simulink model "intel_motor_control_rl2freddie"  (Simulink 10.3)
settings: Solver=FixedStepDiscrete  StartTime=0.0  StopTime=0.7  FixedStep=62.5e-6 % 16 kHz  RelTol=1e-3  EnableMultiTasking=on
undefined symbols (not defined in the file or in its folder): DiscIntNeverNeededParam, I_max, Position_PI_Limit
libraries: simulink x9, dspsrcs4 x2, rllib x1
(part 1 of 2)
settings Model: Creator=tchau  LastModifiedBy=ludwigjonsson  MultithreadedSim=on
settings Model: SuppressorTable=|
  | <?xml version="1.0" encoding="UTF-8" standalone="yes" ?>
  | <!DOCTYPE boost_serialization>
  | <boost_serialization signature="serialization::archive" version="17">
  | <DiagnosticSuppressor class_id="0" tracking_level="0" version="7">
  | 	<Table class_id="1" tracking_level="0" version="0">
  | 		<count>1</count>
  | 		<bucket_count>2</bucket_count>
  | 		<item_version>0</item_version>
  | 		<item class_id="2" tracking_level="0" version="0">
  | 			<first class_id="3" tracking_level="0" version="7">
  | 				<Source class_id="4" tracking_level="0" version="0">
  | 					<count>1</count>
  | 					<item_version>0</item_version>
  | 					<item>7415:2</item>
  | 				</Source>
  | 			</first>
  | 			<second class_id="5" tracking_level="0" version="7">
  | 				<SuppressedData class_id="6" tracking_level="0" version="0">
  | 					<count>2</count>
  | 					<bucket_count>2</bucket_count>
  | 					<item_version>0</item_version>
  | 					<item class_id="7" tracking_level="0" version="0">
  | 						<first class_id="8" tracking_level="0" version="7">
  | 							<ID>Simulink:DataType:WarningOverFlowDetected</ID>
  | 							<Cause>
  | 								<Source>
  | 									<count>0</count>
  | 									<item_version>0</item_version>
  | 								</Source>
  | 							</Cause>
  | 						</first>
  | 						<second class_id="9" tracking_level="0" version="7">
  | 							<Comment></Comment>
  | 							<User></User>
  | 							<LastModified class_id="10" tracking_level="0" version="0">
  | 								<ptime_date class_id="11" tracking_level="0" version="0">
  | 									<date>20160608</date>
  | 								</ptime_date>
  | 								<ptime_time_duration class_id="12" tracking_level="0" version="1">
  | 									<is_special>0</is_special>
  | 									<time_duration_hours>15</time_duration_hours>
  | 									<time_duration_minutes>23</time_duration_minutes>
  | 									<time_duration_seconds>17</time_duration_seconds>
  | 									<time_duration_fractional_seconds>0</time_duration_fractional_seconds>
  | 								</ptime_time_duration>
  | 							</LastModified>
  | 							<SuppressionType>1</SuppressionType>
  | 						</second>
  | 					</item>
  | 					<item>
  | 						<first>
  | 							<ID>SimulinkFixedPoint:util:Overflowoccurred</ID>
  | 							<Cause>
  | 								<Source>
  | 									<count>0</count>
  | 									<item_version>0</item_version>
  | 								</Source>
  | 							</Cause>
  | 						</first>
  | 						<second>
  | 							<Comment></Comment>
  | 							<User></User>
  | 							<LastModified>
  | 								<ptime_date>
  | 									<date>20160608</date>
  | 								</ptime_date>
  | 								<ptime_time_duration>
  | 									<is_special>0</is_special>
  | 									<time_duration_hours>15</time_duration_hours>
  | 									<time_duration_minutes>23</time_duration_minutes>
  | 									<time_duration_seconds>17</time_duration_seconds>
  | 									<time_duration_fractional_seconds>0</time_duration_fractional_seconds>
  | 								</ptime_time_duration>
  | 							</LastModified>
  | 							<SuppressionType>1</SuppressionType>
  | 						</second>
  | 					</item>
  | 				</SuppressedData>
  | 			</second>
  | 		</item>
  | 	</Table>
  | </DiagnosticSuppressor>
  | 
  | </boost_serialization>
  | 
  | </boost_serialization>
settings DataIOCC: SignalLoggingSaveFormat=Dataset  SaveOutput=off  SignalLogging=off  DSMLogging=off  SaveTime=off  ReturnWorkspaceOutputs=on
settings OptimizationCC: BlockReduction=off  ConditionallyExecuteInputs=off  DefaultParameterBehavior=Inlined  InlineInvariantSignals=on  ExpressionDepthLimit=128  EfficientFloat2IntCast=on  SimCompilerOptimization=on
settings DebuggingCC: AlgebraicLoopMsg=error  UnderspecifiedInitializationDetection=Simplified  MergeDetectMultiDrivingBlocksExec=error  SolverPrmCheckMsg=warning  SingleTaskRateTransMsg=error  FcnCallInpInsideContextMsg=error  StateNameClashWarn=none
settings HardwareCC: ProdHWDeviceType=ASIC/FPGA->ASIC/FPGA  TargetBitPerLong=64  TargetBitPerPointer=64  TargetBitPerSizeT=64  TargetBitPerPtrDiffT=64  TargetLongLongMode=on  TargetIntDivRoundTo=Zero  TargetEndianess=LittleEndian  TargetWordSize=64  TargetHWDeviceType=MATLAB Host  ProdEqTarget=off
settings GRTTargetCC: CombineOutputUpdateFcns=on  MatFileLogging=off  SupportNonFinite=off  GRTInterface=off

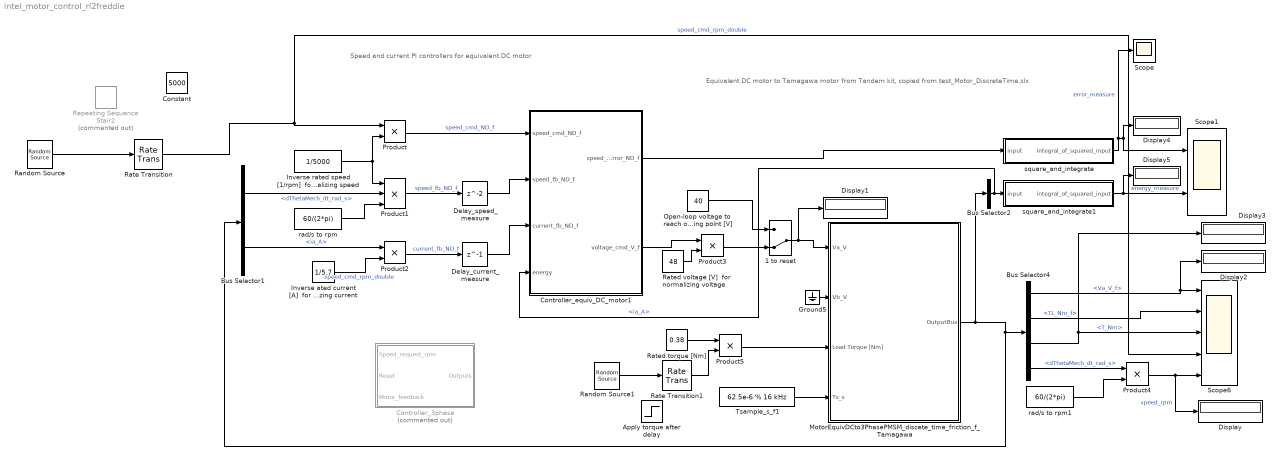
== system intel_motor_control_rl2freddie ==
  note: Equivalent DC motor to Tamagawa motor from Tandem kit,
      | copied from test_Motor_DiscreteTime.slx
  note: Speed and current PI controllers
      | for equivalent DC motor
  1 to reset : ManualSwitch  CurrentSetting=0
  "Apply torque after delay " : Step  Time=0.05  SampleTime=0
  Bus Selector1 : BusSelector  OutputSignals=dThetaMech_dt_rad_s,ia_A
  Bus Selector2 : BusSelector  OutputSignals=ia_A
  Bus Selector4 : BusSelector  OutputSignals=Va_V_f,TL_Nm_f,T_Nm,dThetaMech_dt_rad_s
  Constant : Constant  Value=5000
  Controller_3phase : Subsystem  Commented=on
  Controller_equiv_DC_motor1 : Subsystem
  Delay_current_measure : Delay  DelayLength=1  InitialCondition=0
  Delay_speed_measure : Delay  InitialCondition=0
  Display{,1..5} (6 alike) : Display
  Ground5 : Ground
  Inverse ated current [A]  for normalizing current : Constant  Value=1/5.7  OutDataTypeStr=double
  Inverse rated speed [1/rpm]  for normalizing speed : Constant  Value=1/5000  OutDataTypeStr=double
  MotorEquivDCto3PhasePMSM_discete_time_friction_f_Tamagawa : Subsystem  mask(Intel PMSM equiv DC){R_ohm=0.68/3, L_H=3e-3/3, Ke_Vs_rad=0.07, Kt_Nm_A=0.07, PolePairs_int=2, J_kgm2=0.165e-4, Tf_Nm=0.02}
      mask prompts: R_ohm "Phase resistance [Ohm]"; L_H "Phase inductance [H]"; Ke_Vs_rad "Back-emf constant kE, based on peak phase values [Vs/rad]"; Kt_Nm_A "Motor torque constant kT, based on peak phase values [Nm/A]"; PolePairs_int "Number of pole pairs (0.5*n poles)  [integer]"; J_kgm2 "Mechanical inertia [kgm^2]"; Tf_Nm "Static friction Tf [Nm]"
      mask help: Intel motor model, equiv DC to PMSM
  Open-loop voltage to  reach operating point [V] : Constant  Value=40  OutDataTypeStr=double
  Product{,2..5} (5 alike) : Product
  Product1 : Product  Inputs=***
  Random Source : dspsrcs4/Random Source  SrcType=Uniform  NormMethod=Ziggurat  CltLength=12  MinVal=-5000  MaxVal=5000  MeanVal=0  VarVal=1  RepMode=Specify seed  rawSeed=randSeed  IsInherit=off  SampMode=Discrete  SampTime=650*62.5e-6  SampFrame=1  DataType=Double  OutComplex=Real  OutputFrames=off
  Random Source1 : dspsrcs4/Random Source  SrcType=Uniform  NormMethod=Ziggurat  CltLength=12  MinVal=-1  MaxVal=1  MeanVal=0  VarVal=1  RepMode=Specify seed  rawSeed=randSeed  IsInherit=off  SampMode=Discrete  SampTime=450*62.5e-6  SampFrame=1  DataType=Double  OutComplex=Real  OutputFrames=off
  Rate Transition : RateTransition  OutPortSampleTime=62.5e-6
  Rate Transition1 : RateTransition  OutPortSampleTime=62.5e-6
  Rated torque [Nm] : Constant  Value=0.38  OutDataTypeStr=double
  Rated voltage [V]  for normalizing voltage : Constant  Value=48  OutDataTypeStr=double
  Repeating Sequence Stair2 : simulink/Sources/Repeating Sequence Stair  Commented=on  OutValues=(rand(200,1)-0.5)*10000  tsamp=500*62.5e-6  OutMin=[]  OutMax=[]  OutDataTypeStr=double  OutputDataTypeScalingMode=double  OutDataType=fixdt(0,8)  ConRadixGroup=Best Precision: Vector-wise  OutScaling=2^-12
  Scope : Scope
  Scope1 : Scope  NumInputPorts=2
  Scope6 : Scope  NumInputPorts=5
  Tsample_s_f1 : Constant  Value=62.5e-6 % 16 kHz  OutDataTypeStr=double
  rad/s to rpm : Constant  Value=60/(2*pi)  OutDataTypeStr=double
  rad/s to rpm1 : Constant  Value=60/(2*pi)  OutDataTypeStr=double
  square_and_integrate : Subsystem
  square_and_integrate1 : Subsystem
  wires:
  Rate Transition/1 -> Scope6/4, Product/1  "speed_cmd_rpm_double"
  MotorEquivDCto3PhasePMSM_discete_time_friction_f_Tamagawa/1(OutputBus) -> Bus Selector2/1, Bus Selector1/1, Bus Selector4/1
  Bus Selector4/3 -> Scope6/3, Display3/1  "<T_Nm>"
  Ground5/1 -> MotorEquivDCto3PhasePMSM_discete_time_friction_f_Tamagawa/2(Vb_V)
  Bus Selector4/1 -> Display2/1, Scope6/1  "<Va_V_f>"
  Product5/1 -> MotorEquivDCto3PhasePMSM_discete_time_friction_f_Tamagawa/3(Load Torque [Nm])
  Bus Selector4/4 -> Product4/1  "<dThetaMech_dt_rad_s>"
  Product/1 -> Controller_equiv_DC_motor1/1(speed_cmd_ND_f)  "speed_cmd_ND_f"
  Tsample_s_f1/1 -> MotorEquivDCto3PhasePMSM_discete_time_friction_f_Tamagawa/4(Ts_s)
  Inverse rated speed [1/rpm]  for normalizing speed/1 -> Product1/1, Product/2
  Product1/1 -> Delay_speed_measure/1  "speed_fb_ND_f"
  Bus Selector1/1 -> Product1/2  "<dThetaMech_dt_rad_s>"
  Bus Selector1/2 -> Product2/1  "<ia_A>"
  Inverse ated current [A]  for normalizing current/1 -> Product2/2  "speed_cmd_rpm_double"
  Controller_equiv_DC_motor1/2(voltage_cmd_V_f) -> Product3/1
  Rated voltage [V]  for normalizing voltage/1 -> Product3/2
  rad/s to rpm/1 -> Product1/3
  Product2/1 -> Delay_current_measure/1  "current_fb_ND_f"
  Product4/1 -> Scope6/5, Display/1  "speed_rpm"
  rad/s to rpm1/1 -> Product4/2
  Open-loop voltage to  reach operating point [V]/1 -> 1 to reset/1
  Product3/1 -> 1 to reset/2
  1 to reset/1 -> Display1/1, MotorEquivDCto3PhasePMSM_discete_time_friction_f_Tamagawa/1(Va_V)
  Rated torque [Nm]/1 -> Product5/1
  Bus Selector4/2 -> Scope6/2  "<TL_Nm_f>"
  Controller_equiv_DC_motor1/1(speed_error_ND_f) -> square_and_integrate/1(input)
  square_and_integrate/1(integral_of_squared_input) -> Scope/1, Scope1/1, Display4/1  "error_measure"
  Bus Selector2/1 -> Controller_equiv_DC_motor1/4(energy), square_and_integrate1/1(input)  "<ia_A>"
  square_and_integrate1/1(integral_of_squared_input) -> Display5/1, Scope1/2  "energy_measure"
  Delay_speed_measure/1 -> Controller_equiv_DC_motor1/2(speed_fb_ND_f)
  Delay_current_measure/1 -> Controller_equiv_DC_motor1/3(current_fb_ND_f)
  Random Source1/1 -> Rate Transition1/1
  Random Source/1 -> Rate Transition/1
  Rate Transition1/1 -> Product5/2

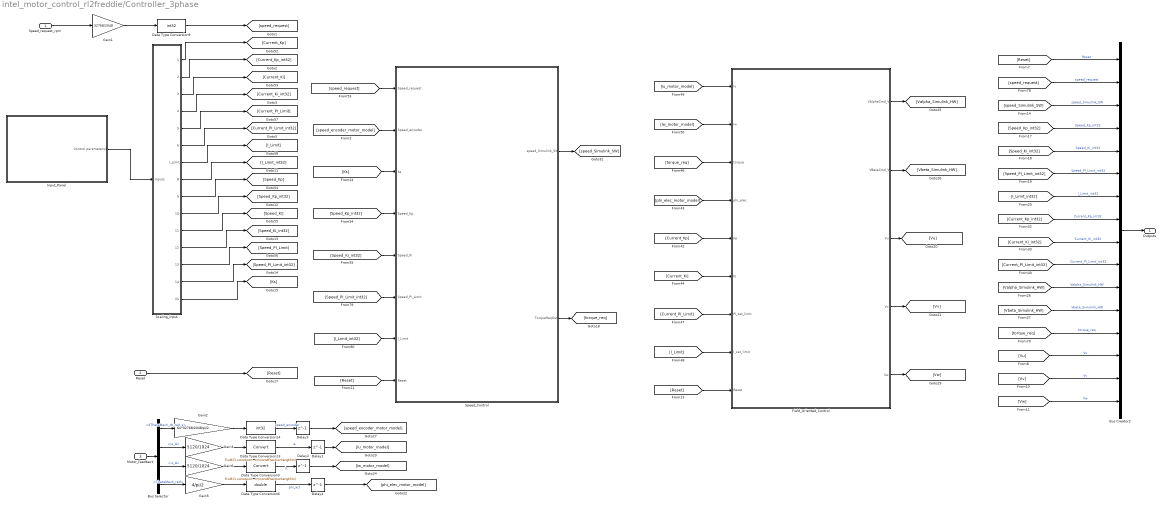
== system intel_motor_control_rl2freddie/Controller_3phase ==
  Speed_request_rpm : Inport
  Reset : Inport  Port=2  PortDimensions=1
  Motor_feedback : Inport  Port=3
  Bus Creator2 : BusCreator  Inputs=16
  Bus Selector : BusSelector  OutputSignals=dThetaMech_dt_rad_s,ia_A,ic_A,ThetaMech_rad
  Data Type Conversion13 : DataTypeConversion  OutDataTypeStr=fixdt(1,constwordlengthIn,constfractionlengthIn)
  Data Type Conversion14 : DataTypeConversion  OutDataTypeStr=int32
  Data Type Conversion3 : DataTypeConversion  OutDataTypeStr=fixdt(1,constwordlengthIn,constfractionlengthIn)
  Data Type Conversion6 : DataTypeConversion  OutDataTypeStr=double
  Data Type Conversion9 : DataTypeConversion  OutDataTypeStr=int32
  Delay{1..4} (4 alike) : Delay  DelayLength=1  InitialCondition=0
  Field_Oriented_Control : Subsystem
  Gain1 : Gain  Gain=32768/2048
  Gain2 : Gain  Gain=60*32768/2048/pi/2  OutDataTypeStr=single
  Gain3 : Gain  Gain=5120/1024  OutDataTypeStr=single
  Gain5 : Gain  Gain=4/pi/2  OutDataTypeStr=single
  Gain6 : Gain  Gain=5120/1024  OutDataTypeStr=single
  Input_Panel : Subsystem
      mask Display: fprintf('Setup\nParameters')
  Scaling_input : Subsystem
  Speed_Control : Subsystem
  Outputs : Outport
  wires:
  Data Type Conversion9/1 -> [speed_request]
  Speed_request_rpm/1 -> Gain1/1
  Gain1/1 -> Data Type Conversion9/1
  Input_Panel/1(Control parameters1) -> Scaling_input/1(Inputs)
  Field_Oriented_Control/2(VBetaCmd_V) -> [Vbeta_Simulink_HW]
  Field_Oriented_Control/1(VAlphaCmd_V) -> [Valpha_Simulink_HW]
  Data Type Conversion3/1 -> Delay2/1  "ic"
  Gain6/1 -> Data Type Conversion3/1
  Data Type Conversion13/1 -> Delay1/1  "ia"
  Gain3/1 -> Data Type Conversion13/1
  Data Type Conversion6/1 -> Delay4/1  "phi_act"
  Gain5/1 -> Data Type Conversion6/1
  Data Type Conversion14/1 -> Delay3/1  "speed_encoder"
  Gain2/1 -> Data Type Conversion14/1
  [Vw] -> Bus Creator2/16  "Vw"
  [Vv] -> Bus Creator2/15  "Vv"
  [Vu] -> Bus Creator2/14  "Vu"
  Field_Oriented_Control/5(Vw) -> [Vw]
  Bus Selector/2 -> Gain3/1  "<ia_A>"
  Bus Selector/4 -> Gain5/1  "<ThetaMech_rad>"
  Bus Selector/1 -> Gain2/1  "<dThetaMech_dt_rad_s>"
  Delay3/1 -> [speed_encoder_motor_model]
  Bus Selector/3 -> Gain6/1  "<ic_A>"
  Delay4/1 -> [phi_elec_motor_model]
  Delay2/1 -> [Iw_motor_model]
  Delay1/1 -> [Iu_motor_model]
  [speed_encoder_motor_model] -> Speed_Control/2(Speed_encoder)
  Motor_feedback/1 -> Bus Selector/1
  Field_Oriented_Control/4(Vv) -> [Vv]
  Field_Oriented_Control/3(Vu) -> [Vu]
  [Reset] -> Field_Oriented_Control/9(Reset)
  [I_Limit] -> Field_Oriented_Control/8(I_sat_limit)
  [Current_PI_Limit] -> Field_Oriented_Control/7(PI_sat_limit)
  [Current_Ki] -> Field_Oriented_Control/6(Ki)
  [Current_Kp] -> Field_Oriented_Control/5(Kp)
  [phi_elec_motor_model] -> Field_Oriented_Control/4(phi_elec)
  [torque_req] -> Field_Oriented_Control/3(torque)
  [Iw_motor_model] -> Field_Oriented_Control/2(Iw)
  [Iu_motor_model] -> Field_Oriented_Control/1(Iu)
  [torque_req] -> Bus Creator2/13  "torque_req"
  [Vbeta_Simulink_HW] -> Bus Creator2/12  "Vbeta_Simulink_HW"
  [Valpha_Simulink_HW] -> Bus Creator2/11  "Valpha_Simulink_HW"
  Bus Creator2/1 -> Outputs/1
  [Reset] -> Bus Creator2/1  "Reset"
  [Current_PI_Limit_int32] -> Bus Creator2/10  "Current_PI_Limit_int32"
  [Current_Ki_int32] -> Bus Creator2/9  "Current_Ki_int32"
  [Current_Kp_int32] -> Bus Creator2/8  "Current_Kp_int32"
  [I_Limit_int32] -> Bus Creator2/7  "I_Limit_int32"
  [Speed_PI_Limit_int32] -> Bus Creator2/6  "Speed_PI_Limit_int32"
  [Speed_Ki_int32] -> Bus Creator2/5  "Speed_Ki_int32"
  [Speed_Kp_int32] -> Bus Creator2/4  "Speed_Kp_int32"
  [I_Limit_int32] -> Speed_Control/7(I_Limit)
  [Speed_PI_Limit_int32] -> Speed_Control/6(Speed_PI_Limit)
  [Speed_Ki_int32] -> Speed_Control/5(Speed_Ki)
  [Speed_Kp_int32] -> Speed_Control/4(Speed_Kp)
  [speed_request] -> Speed_Control/1(Speed_request)
  Scaling_input/15(Ks) -> [Ks]
  Scaling_input/14(Speed_PI_Limit_int32) -> [Speed_PI_Limit_int32]
  Scaling_input/13(Speed_PI_Limit) -> [Speed_PI_Limit]
  Scaling_input/12(Speed_Ki_int32) -> [Speed_Ki_int32]
  Scaling_input/11(Speed_Ki) -> [Speed_Ki]
  Scaling_input/10(Speed_Kp_int32) -> [Speed_Kp_int32]
  Scaling_input/9(Speed_Kp) -> [Speed_Kp]
  Scaling_input/8(I_Limit_int32) -> [I_Limit_int32]
  Scaling_input/7(I_Limit) -> [I_Limit]
  Scaling_input/6(Current_PI_Limit_int32) -> [Current_PI_Limit_int32]
  Scaling_input/5(Current_PI_Limit) -> [Current_PI_Limit]
  Scaling_input/4(Current_Ki_int32) -> [Current_Ki_int32]
  Scaling_input/3(Current_Ki) -> [Current_Ki]
  Scaling_input/2(Current_Kp_int32) -> [Current_Kp_int32]
  Scaling_input/1(Current_Kp) -> [Current_Kp]
  [speed_request] -> Bus Creator2/2  "speed_request"
  Reset/1 -> [Reset]
  [speed_Simulink_SW] -> Bus Creator2/3  "speed_Simulink_SW"
  [Ks] -> Speed_Control/3(Ks)
  [Reset] -> Speed_Control/8(Reset)
  Speed_Control/1(speed_Simulink_SW) -> [speed_Simulink_SW]
  Speed_Control/2(TorqueReqOut) -> [torque_req]

== system intel_motor_control_rl2freddie/Controller_equiv_DC_motor1 ==
  note: RL Controller
  speed_cmd_ND_f : Inport
  speed_fb_ND_f : Inport  Port=2  PortDimensions=1
  current_fb_ND_f : Inport  Port=3  PortDimensions=1
  energy : Inport  Port=4
  1 to reset : ManualSwitch
  FALSE_bool : Constant  Value=0  OutDataTypeStr=boolean
  PI_Ctrl_float_speed : Subsystem
  TRUE_bool : Constant  OutDataTypeStr=boolean
  abs_limit_output_ND_f : Constant  OutDataTypeStr=double
  speed_error_ND_f : Outport
  voltage_cmd_V_f : Outport  Port=2
  wires:
  speed_cmd_ND_f/1 -> PI_Ctrl_float_speed/1(cmd_f)
  speed_fb_ND_f/1 -> PI_Ctrl_float_speed/2(fb_f)
  abs_limit_output_ND_f/1 -> PI_Ctrl_float_speed/3(output_abs_limit_f)
  current_fb_ND_f/1 -> PI_Ctrl_float_speed/6(Icurrent_fb)
  1 to reset/1 -> PI_Ctrl_float_speed/4(Reset_bool)
  FALSE_bool/1 -> 1 to reset/1
  TRUE_bool/1 -> 1 to reset/2
  PI_Ctrl_float_speed/1(error_f) -> speed_error_ND_f/1  "speed_error_ND_f"
  energy/1 -> PI_Ctrl_float_speed/5(energy)
  PI_Ctrl_float_speed/2(output_f) -> voltage_cmd_V_f/1

== system intel_motor_control_rl2freddie/MotorEquivDCto3PhasePMSM_discete_time_friction_f_Tamagawa ==
  Va_V : Inport
  Vb_V : Inport  Port=2
  Load Torque [Nm] : Inport  Port=3
  Ts_s : Inport  Port=4
  Bus Creator1 : BusCreator  Inputs=7
  Load Torque [Nm]1 : InportShadow  Port=3
  Motor electromagnetic : Subsystem
  Motor mechanical : Subsystem  mask(Inertia){J_kgm2=J_kgm2}
      mask prompts: J_kgm2 "Inertia [kgm^2]"
      mask help:
      | Mechanical inertia with two attachment points A and B.
      | Torque is applied to the inertia from side A and side B.
      | The combined torque acting on the inertia produces acceleration,
      | velocity and displacement. Velocity and displacement are output as these
      | are the states of the system.
  Ts_s1 : InportShadow  Port=4
  Va_V1 : InportShadow
  Vb_V1 : InportShadow  Port=2
  OutputBus : Outport
  wires:
  Ts_s1/1 -> Motor electromagnetic/4(Ts_s)
  Motor mechanical/1(dTheta_dt_rad_s) -> Motor electromagnetic/3(dThetaMech_dt_rad_s), Bus Creator1/6  "dThetaMech_dt_rad_s"
  Ts_s/1 -> Motor mechanical/3(Ts_s)
  Load Torque [Nm]/1 -> Motor mechanical/2(TB_Nm)  "TL_Nm_f"
  Va_V/1 -> Motor electromagnetic/1(Va_V)  "Va_V_f"
  Bus Creator1/1 -> OutputBus/1
  Vb_V/1 -> Motor electromagnetic/2(Vb_V)  "Vb_V_f"
  Va_V1/1 -> Bus Creator1/1  "Va_V_f"
  Vb_V1/1 -> Bus Creator1/2  "Vb_V_f"
  Motor electromagnetic/1(ia_A) -> Bus Creator1/4  "ia_A"
  Motor electromagnetic/2(T_Nm) -> Motor mechanical/1(TA_Nm), Bus Creator1/5  "T_Nm"
  Motor mechanical/2(Theta_rad) -> Bus Creator1/7  "ThetaMech_rad"
  Load Torque [Nm]1/1 -> Bus Creator1/3  "TL_Nm_f"

== system intel_motor_control_rl2freddie/square_and_integrate ==
  input : Inport
  Add : Sum
  Product6 : Product  Inputs=***
  Tsample_s_f2 : Constant  Value=62.5e-6 % 16 kHz  OutDataTypeStr=double
  delay_to_integrate : Delay  DelayLength=1  InitialCondition=0
  integral_of_squared_input : Outport
  wires:
  delay_to_integrate/1 -> integral_of_squared_input/1, Add/2
  Product6/1 -> Add/1
  Tsample_s_f2/1 -> Product6/3
  Add/1 -> delay_to_integrate/1
  input/1 -> Product6/1, Product6/2

== system intel_motor_control_rl2freddie/square_and_integrate1 ==
  input : Inport
  Add : Sum
  Product6 : Product  Inputs=***
  Tsample_s_f2 : Constant  Value=62.5e-6 % 16 kHz  OutDataTypeStr=double
  delay_to_integrate : Delay  DelayLength=1  InitialCondition=0
  integral_of_squared_input : Outport
  wires:
  input/1 -> Product6/2, Product6/1
  Add/1 -> delay_to_integrate/1
  Tsample_s_f2/1 -> Product6/3
  Product6/1 -> Add/1
  delay_to_integrate/1 -> Add/2, integral_of_squared_input/1

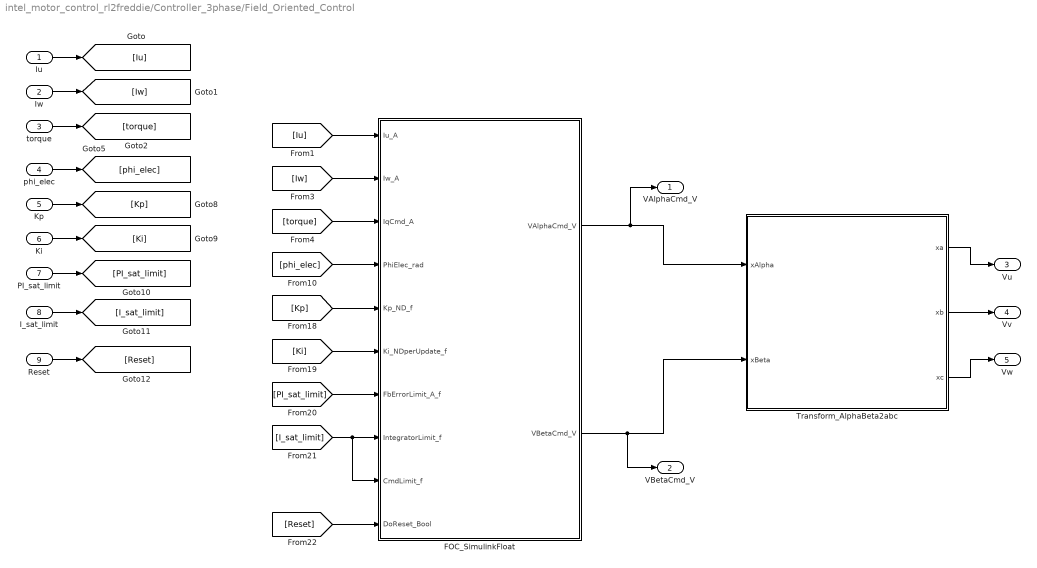
== system intel_motor_control_rl2freddie/Controller_3phase/Field_Oriented_Control ==
  Iu : Inport
  Iw : Inport  Port=2
  torque : Inport  Port=3
  phi_elec : Inport  Port=4
  Kp : Inport  Port=5
  Ki : Inport  Port=6
  PI_sat_limit : Inport  Port=7
  I_sat_limit : Inport  Port=8
  Reset : Inport  Port=9
  FOC_SimulinkFloat : Subsystem
  Transform_AlphaBeta2abc : Subsystem  mask(Transform_AlphaBeta2abc){}
      mask help:
      | Transformation from equivalent Alpha-Beta 2-phase stator-based values to original 3-phase stator coil values.
      | Scaling chosen so peak values remain the same.
      mask Help:
      | Transformation from equivalent Alpha-Beta 2-phase stator-based values to original 3-phase stator coil values.
      | Scaling chosen so peak values remain the same.
      | Transformation equations:
      | 
      | xa = xAlpha
      | xb = -0.5*xAlpha + 0.5*sqrt(3)*xBeta
      | xc = -0.5*xAlpha - 0.5*sqrt(3)*xBeta
      mask Display:
      | port_label('output', 1, 'xa')
      | port_label('output', 2, 'xb')
      | port_label('output', 3, 'xc')
      | port_label('input', 1, 'xAlpha')
      | port_label('input', 2, 'xBeta')
      | disp ('xa=xAlpha\nxb=-0.5*xAlpha+0.5*sqrt(3)*xBeta\nxc=-0.5*xAlpha-0.5*sqrt(3)*xBeta');
  VAlphaCmd_V : Outport
  VBetaCmd_V : Outport  Port=2
  Vu : Outport  Port=3
  Vv : Outport  Port=4
  Vw : Outport  Port=5
  wires:
  Transform_AlphaBeta2abc/3(xc) -> Vw/1
  Transform_AlphaBeta2abc/1(xa) -> Vu/1
  Transform_AlphaBeta2abc/2(xb) -> Vv/1
  [Reset] -> FOC_SimulinkFloat/10(DoReset_Bool)
  [I_sat_limit] -> FOC_SimulinkFloat/8(IntegratorLimit_f), FOC_SimulinkFloat/9(CmdLimit_f)
  [PI_sat_limit] -> FOC_SimulinkFloat/7(FbErrorLimit_A_f)
  [Ki] -> FOC_SimulinkFloat/6(Ki_NDperUpdate_f)
  [Kp] -> FOC_SimulinkFloat/5(Kp_ND_f)
  Reset/1 -> [Reset]
  I_sat_limit/1 -> [I_sat_limit]
  PI_sat_limit/1 -> [PI_sat_limit]
  Ki/1 -> [Ki]
  Kp/1 -> [Kp]
  [phi_elec] -> FOC_SimulinkFloat/4(PhiElec_rad)
  phi_elec/1 -> [phi_elec]
  [torque] -> FOC_SimulinkFloat/3(IqCmd_A)
  torque/1 -> [torque]
  Iw/1 -> [Iw]
  [Iw] -> FOC_SimulinkFloat/2(Iw_A)
  [Iu] -> FOC_SimulinkFloat/1(Iu_A)
  Iu/1 -> [Iu]
  FOC_SimulinkFloat/2(VBetaCmd_V) -> Transform_AlphaBeta2abc/2(xBeta), VBetaCmd_V/1
  FOC_SimulinkFloat/1(VAlphaCmd_V) -> Transform_AlphaBeta2abc/1(xAlpha), VAlphaCmd_V/1

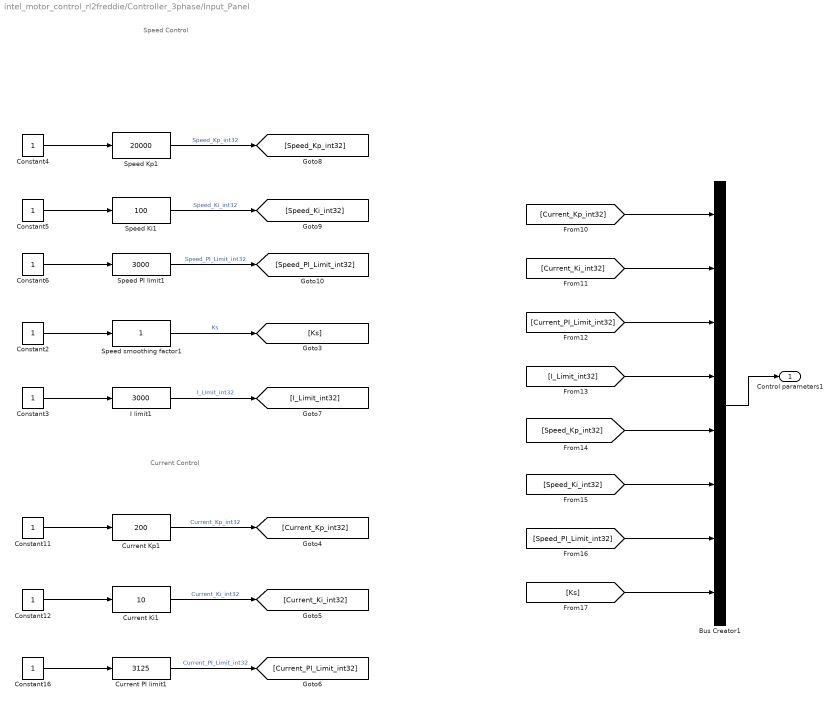
== system intel_motor_control_rl2freddie/Controller_3phase/Input_Panel ==
  note: Current Control
  note: Speed Control
  Bus Creator1 : BusCreator  Inputs=8
  Constant{3..6,11..12,16} (7 alike) : Constant  OutDataTypeStr=int32
  Constant2 : Constant  OutDataTypeStr=fixdt(0,16,15)
  Current Ki1 : simulink/Math Operations/Slider Gain  gain=10  low=0  high=100
  Current Kp1 : simulink/Math Operations/Slider Gain  gain=200  low=0  high=1000
  Current PI limit1 : simulink/Math Operations/Slider Gain  gain=3125  low=0  high=10000
  I limit1 : simulink/Math Operations/Slider Gain  gain=3000  low=0  high=10000
  Speed Ki1 : simulink/Math Operations/Slider Gain  gain=100  low=0  high=1000
  Speed Kp1 : simulink/Math Operations/Slider Gain  gain=20000  low=0  high=100000
  Speed PI limit1 : simulink/Math Operations/Slider Gain  gain=3000  low=0  high=10000
  Speed smoothing factor1 : simulink/Math Operations/Slider Gain  gain=1  low=0  high=1
  Control parameters1 : Outport
  wires:
  [Current_Kp_int32] -> Bus Creator1/1
  [Current_Ki_int32] -> Bus Creator1/2
  [Current_PI_Limit_int32] -> Bus Creator1/3
  [I_Limit_int32] -> Bus Creator1/4
  [Speed_Kp_int32] -> Bus Creator1/5
  [Speed_Ki_int32] -> Bus Creator1/6
  [Speed_PI_Limit_int32] -> Bus Creator1/7
  [Ks] -> Bus Creator1/8
  Constant3/1 -> I limit1/1
  Constant16/1 -> Current PI limit1/1
  Constant12/1 -> Current Ki1/1
  Constant11/1 -> Current Kp1/1
  I limit1/1 -> [I_Limit_int32]  "I_Limit_int32"
  Current PI limit1/1 -> [Current_PI_Limit_int32]  "Current_PI_Limit_int32"
  Current Ki1/1 -> [Current_Ki_int32]  "Current_Ki_int32"
  Current Kp1/1 -> [Current_Kp_int32]  "Current_Kp_int32"
  Constant6/1 -> Speed PI limit1/1
  Constant5/1 -> Speed Ki1/1
  Constant4/1 -> Speed Kp1/1
  Speed PI limit1/1 -> [Speed_PI_Limit_int32]  "Speed_PI_Limit_int32"
  Speed Ki1/1 -> [Speed_Ki_int32]  "Speed_Ki_int32"
  Speed Kp1/1 -> [Speed_Kp_int32]  "Speed_Kp_int32"
  Speed smoothing factor1/1 -> [Ks]  "Ks"
  Constant2/1 -> Speed smoothing factor1/1
  Bus Creator1/1 -> Control parameters1/1

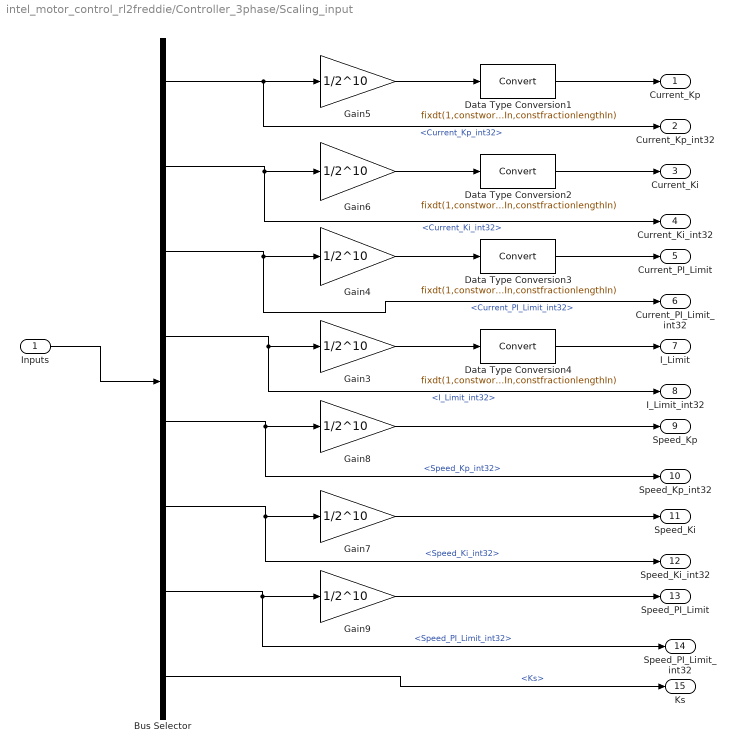
== system intel_motor_control_rl2freddie/Controller_3phase/Scaling_input ==
  Inputs : Inport
  Bus Selector : BusSelector  OutputSignals=Current_Kp_int32,Current_Ki_int32,Current_PI_Limit_int32,I_Limit_int32,Speed_Kp_int32,Speed_Ki_int32,Speed_PI_Limit_int32,Ks
  Data Type Conversion{1..4} (4 alike) : DataTypeConversion  OutDataTypeStr=fixdt(1,constwordlengthIn,constfractionlengthIn)
  Gain{3..9} (7 alike) : Gain  Gain=1/2^10  OutDataTypeStr=single
  Current_Kp : Outport
  Current_Kp_int32 : Outport  Port=2
  Current_Ki : Outport  Port=3
  Current_Ki_int32 : Outport  Port=4
  Current_PI_Limit : Outport  Port=5
  Current_PI_Limit_int32 : Outport  Port=6
  I_Limit : Outport  Port=7
  I_Limit_int32 : Outport  Port=8
  Speed_Kp : Outport  Port=9
  Speed_Kp_int32 : Outport  Port=10
  Speed_Ki : Outport  Port=11
  Speed_Ki_int32 : Outport  Port=12
  Speed_PI_Limit : Outport  Port=13
  Speed_PI_Limit_int32 : Outport  Port=14
  Ks : Outport  Port=15
  wires:
  Gain4/1 -> Data Type Conversion3/1
  Bus Selector/3 -> Gain4/1, Current_PI_Limit_int32/1  "<Current_PI_Limit_int32>"
  Bus Selector/4 -> Gain3/1, I_Limit_int32/1  "<I_Limit_int32>"
  Gain7/1 -> Speed_Ki/1
  Gain6/1 -> Data Type Conversion2/1
  Gain3/1 -> Data Type Conversion4/1
  Gain5/1 -> Data Type Conversion1/1
  Data Type Conversion4/1 -> I_Limit/1
  Data Type Conversion1/1 -> Current_Kp/1
  Inputs/1 -> Bus Selector/1
  Data Type Conversion2/1 -> Current_Ki/1
  Gain9/1 -> Speed_PI_Limit/1
  Bus Selector/2 -> Gain6/1, Current_Ki_int32/1  "<Current_Ki_int32>"
  Bus Selector/1 -> Gain5/1, Current_Kp_int32/1  "<Current_Kp_int32>"
  Data Type Conversion3/1 -> Current_PI_Limit/1
  Bus Selector/8 -> Ks/1  "<Ks>"
  Bus Selector/5 -> Gain8/1, Speed_Kp_int32/1  "<Speed_Kp_int32>"
  Bus Selector/7 -> Gain9/1, Speed_PI_Limit_int32/1  "<Speed_PI_Limit_int32>"
  Gain8/1 -> Speed_Kp/1
  Bus Selector/6 -> Gain7/1, Speed_Ki_int32/1  "<Speed_Ki_int32>"

== system intel_motor_control_rl2freddie/Controller_3phase/Speed_Control ==
  note: Speed Estimation
  note: Speed
      | PI Controller
  Speed_request : Inport  PortDimensions=1
  Speed_encoder : Inport  Port=2  PortDimensions=1
  Ks : Inport  Port=3  PortDimensions=1
  Speed_Kp : Inport  Port=4  PortDimensions=1
  Speed_Ki : Inport  Port=5  PortDimensions=1
  Speed_PI_Limit : Inport  Port=6  PortDimensions=1
  I_Limit : Inport  Port=7  PortDimensions=1
  Reset : Inport  Port=8  PortDimensions=1
  Data Type Conversion1 : DataTypeConversion  OutDataTypeStr=int32
  Data Type Conversion2 : DataTypeConversion  OutDataTypeStr=fixdt(1,constwordlength,constfractionlength)
  Data Type Conversion4 : DataTypeConversion  OutDataTypeStr=fixdt(1,constwordlengthIn,constfractionlengthIn)
  Fix_PI_Ctrl_Integ1 : Subsystem
  Gain1 : Gain  Gain=1/2^10
  Gain4 : Gain  Gain=2048/32768  OutDataTypeStr=single
  Speed Filter : Subsystem
  Subtract1 : Sum  Inputs=+-
  speed_Simulink_SW : Outport  PortDimensions=1
  TorqueReqOut : Outport  Port=2  PortDimensions=1
  wires:
  Speed_request/1 -> Subtract1/1
  Speed_encoder/1 -> Speed Filter/1(Velocity)
  Reset/1 -> Fix_PI_Ctrl_Integ1/6(Reset)
  Ks/1 -> Speed Filter/2(Ks)
  Data Type Conversion2/1 -> speed_Simulink_SW/1
  Gain4/1 -> Data Type Conversion2/1
  Gain1/1 -> Data Type Conversion4/1
  Data Type Conversion1/1 -> Fix_PI_Ctrl_Integ1/1(PI_in)
  Fix_PI_Ctrl_Integ1/1(PI_out) -> Gain1/1  "Torque (Nm)"
  Subtract1/1 -> Data Type Conversion1/1
  Speed_Kp/1 -> Fix_PI_Ctrl_Integ1/2(Kp)
  Speed_Ki/1 -> Fix_PI_Ctrl_Integ1/3(Ki)
  Speed_PI_Limit/1 -> Fix_PI_Ctrl_Integ1/4(limit)
  I_Limit/1 -> Fix_PI_Ctrl_Integ1/5(I_max)
  Speed Filter/1(Speed) -> Gain4/1, Subtract1/2
  Data Type Conversion4/1 -> TorqueReqOut/1

== system intel_motor_control_rl2freddie/Controller_equiv_DC_motor1/PI_Ctrl_float_speed ==
  note: Error Input
  cmd_f : Inport
  fb_f : Inport  Port=2
  output_abs_limit_f : Inport  Port=3
  Reset_bool : Inport  Port=4
  energy : Inport  Port=5
  Icurrent_fb : Inport  Port=6
  Constant1 : Constant  Value=0  OutDataTypeStr=Inherit: Inherit via back propagation
  Reinforcement Learning1 : Subsystem
  Subtract1 : Sum  Inputs=+-
  Tanh : Trigonometry  Commented=through  Operator=tanh
  Unit Delay1 : UnitDelay  SampleTime=-1  HasFrameUpgradeWarning=on
  limit_abs_value_of_output : Subsystem
  set_output_to_zero_if_reset : Switch  Criteria=u2 > Threshold
  error_f : Outport
  output_f : Outport  Port=2
  wires:
  output_abs_limit_f/1 -> Reinforcement Learning1/7(abslimit), limit_abs_value_of_output/2(abs_max)
  Tanh/1 -> Unit Delay1/1, set_output_to_zero_if_reset/3
  set_output_to_zero_if_reset/1 -> output_f/1
  Reset_bool/1 -> Reinforcement Learning1/2(isdone), set_output_to_zero_if_reset/2
  Constant1/1 -> set_output_to_zero_if_reset/1
  cmd_f/1 -> Reinforcement Learning1/8(speedin), Subtract1/1
  fb_f/1 -> Subtract1/2, Reinforcement Learning1/4(speedfb)
  Subtract1/1 -> Reinforcement Learning1/1(speederror), error_f/1  "error_f"
  energy/1 -> Reinforcement Learning1/3(energy measure)
  Icurrent_fb/1 -> Reinforcement Learning1/5(cfb)
  Unit Delay1/1 -> Reinforcement Learning1/6(prevact)
  Reinforcement Learning1/1(action) -> limit_abs_value_of_output/1(input)
  limit_abs_value_of_output/1(output) -> Tanh/1

== system intel_motor_control_rl2freddie/MotorEquivDCto3PhasePMSM_discete_time_friction_f_Tamagawa/Motor electromagnetic ==
  note: Single phase to get same rated operating point as 3-phase
  note: Calculate current in phase a.
  Va_V : Inport
  Vb_V : Inport  Port=2
  dThetaMech_dt_rad_s : Inport  Port=3
  Ts_s : Inport  Port=4
  Delay : Delay  DelayLength=1
  Gain_Kt_Nm_A : Gain  Gain=Kt_Nm_A
  Ke_Vs_rad : Gain  Gain=Ke_Vs_rad
  Product : Product
  Sum : Sum  Inputs=|++
  Sum6 : Sum  Inputs=+---
  gain_Ra : Gain  Gain=3*R_ohm
  gain_inverseInductance : Gain  Gain=1/(3*L_H)
  ia_A : Outport
  T_Nm : Outport  Port=2
  wires:
  Ts_s/1 -> Product/2
  Sum/1 -> Delay/1
  Product/1 -> Sum/1
  Delay/1 -> gain_Ra/1, Sum/2, Gain_Kt_Nm_A/1, ia_A/1  "ia_A"
  gain_Ra/1 -> Sum6/4
  gain_inverseInductance/1 -> Product/1  "dia/dt"
  Ke_Vs_rad/1 -> Sum6/3
  Sum6/1 -> gain_inverseInductance/1  "vLa_V"
  Vb_V/1 -> Sum6/2
  dThetaMech_dt_rad_s/1 -> Ke_Vs_rad/1  "dThetaMech_dt_rad_s"
  Gain_Kt_Nm_A/1 -> T_Nm/1  "T_Nm"
  Va_V/1 -> Sum6/1

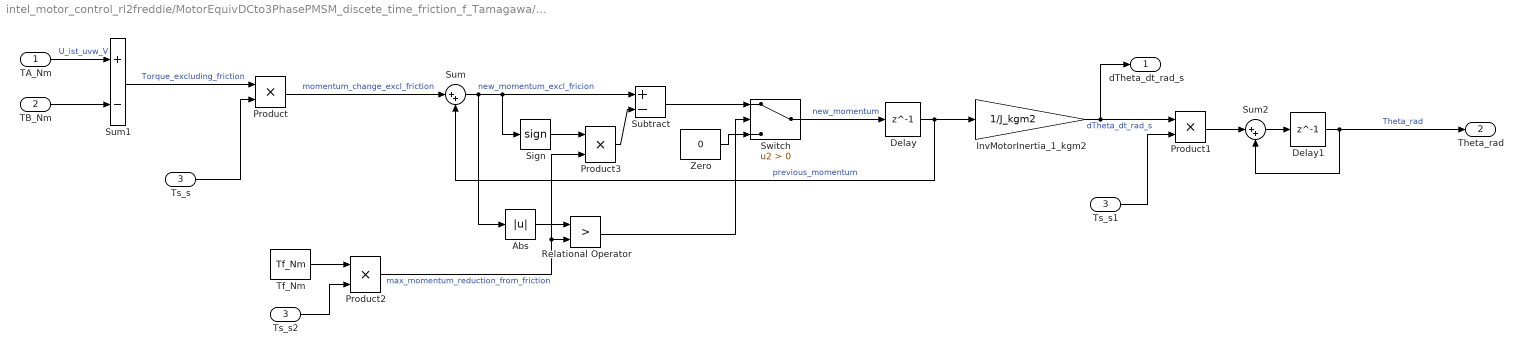
== system intel_motor_control_rl2freddie/MotorEquivDCto3PhasePMSM_discete_time_friction_f_Tamagawa/Motor mechanical ==
  TA_Nm : Inport
  TB_Nm : Inport  Port=2
  Ts_s : Inport  Port=3
  Abs : Abs
  Delay : Delay  DelayLength=1
  Delay1 : Delay  DelayLength=1
  InvMotorInertia_1_kgm2 : Gain  Gain=1/J_kgm2
  Product{,1..3} (4 alike) : Product
  Relational Operator : RelationalOperator  Operator=>  OutDataTypeStr=boolean  RndMeth=Nearest
  Sign : Signum
  Subtract : Sum  Inputs=+-
  Sum : Sum  Inputs=|++
  Sum1 : Sum  Inputs=+-
  Sum2 : Sum  Inputs=|++
  Switch : Switch  Criteria=u2 > Threshold
  Tf_Nm : Constant  Value=Tf_Nm
  Ts_s1 : InportShadow  Port=3
  Ts_s2 : InportShadow  Port=3
  Zero : Constant  Value=0
  dTheta_dt_rad_s : Outport
  Theta_rad : Outport  Port=2
  wires:
  Product1/1 -> Sum2/1
  Sum2/1 -> Delay1/1
  Delay1/1 -> Theta_rad/1, Sum2/2  "Theta_rad"
  Sum/1 -> Abs/1, Sign/1, Subtract/1  "new_momentum_excl_fricion"
  Product/1 -> Sum/1  "momentum_change_excl_friction"
  Ts_s/1 -> Product/2
  Sum1/1 -> Product/1  "Torque_excluding_friction"
  TB_Nm/1 -> Sum1/2
  TA_Nm/1 -> Sum1/1  "U_ist_uvw_V"
  Ts_s1/1 -> Product1/2
  Delay/1 -> InvMotorInertia_1_kgm2/1, Sum/2  "previous_momentum"
  Tf_Nm/1 -> Product2/1
  Ts_s2/1 -> Product2/2
  Product2/1 -> Product3/2, Relational Operator/2  "max_momentum_reduction_from_friction"
  Abs/1 -> Relational Operator/1
  Relational Operator/1 -> Switch/2
  Sign/1 -> Product3/1
  Product3/1 -> Subtract/2
  Subtract/1 -> Switch/1
  Zero/1 -> Switch/3
  Switch/1 -> Delay/1  "new_momentum"
  InvMotorInertia_1_kgm2/1 -> dTheta_dt_rad_s/1, Product1/1  "dTheta_dt_rad_s"

== system intel_motor_control_rl2freddie/Controller_3phase/Field_Oriented_Control/FOC_SimulinkFloat ==
  note: Simulink floating point, based on \depot\ssg\embedded\industrial\MotorControl\ReferenceDesigns\DriveOnChip_SingleIPOneEach_SoC_FFT\SimulinkTests\test_FOC\test_FOC.mdl
  Iu_A : Inport
  Iw_A : Inport  Port=2
  IqCmd_A : Inport  Port=3
  PhiElec_rad : Inport  Port=4
  Kp_ND_f : Inport  Port=5
  Ki_NDperUpdate_f : Inport  Port=6
  FbErrorLimit_A_f : Inport  Port=7
  IntegratorLimit_f : Inport  Port=8
  CmdLimit_f : Inport  Port=9
  DoReset_Bool : Inport  Port=10
  FOC_Simulink_float : Subsystem
  VAlphaCmd_V : Outport
  VBetaCmd_V : Outport  Port=2
  wires:
  FOC_Simulink_float/2(VBetaCmd_V) -> VBetaCmd_V/1
  FOC_Simulink_float/1(VAlphaCmd_V) -> VAlphaCmd_V/1
  DoReset_Bool/1 -> FOC_Simulink_float/10(DoReset_Bool)
  CmdLimit_f/1 -> FOC_Simulink_float/9(CmdLimit_f)
  IntegratorLimit_f/1 -> FOC_Simulink_float/8(IntegratorLimit_f)
  FbErrorLimit_A_f/1 -> FOC_Simulink_float/7(FbErrorLimit_A_f)
  Ki_NDperUpdate_f/1 -> FOC_Simulink_float/6(Ki_NDperUpdate_f)
  Kp_ND_f/1 -> FOC_Simulink_float/5(Kp_ND_f)
  PhiElec_rad/1 -> FOC_Simulink_float/4(PhiElec_rad)
  Iw_A/1 -> FOC_Simulink_float/2(Iw_A)
  Iu_A/1 -> FOC_Simulink_float/1(Iu_A)
  IqCmd_A/1 -> FOC_Simulink_float/3(IqCmd_A)

== system intel_motor_control_rl2freddie/Controller_3phase/Field_Oriented_Control/Transform_AlphaBeta2abc ==
  note: Transformation from equivalent Alpha-Beta 2-phase stator-based values to original 3-phase stator coil values.
      | Scaling chosen so peak values remain the same.
      | Transformation equations:
      |
      | xa = xAlpha
      | xb = -0.5*xAlpha + 0.5*sqrt(3)*xBeta
      | xc = -0.5*xAlpha - 0.5*sqrt(3)*xBeta
  xAlpha : Inport
  xBeta : Inport  Port=2
  Gain1 : Gain  Gain=0.5
  Gain3 : Gain  Gain=sqrt(3)
  Gain5 : Gain  Gain=0.5
  Sum1 : Sum  Inputs=-+
  Sum2 : Sum  Inputs=--
  xa : Outport
  xb : Outport  Port=2
  xc : Outport  Port=3
  wires:
  Gain5/1 -> xb/1
  Sum1/1 -> Gain5/1
  xAlpha/1 -> Sum2/1, Sum1/1, xa/1
  Gain3/1 -> Sum2/2, Sum1/2
  Gain1/1 -> xc/1
  Sum2/1 -> Gain1/1
  xBeta/1 -> Gain3/1

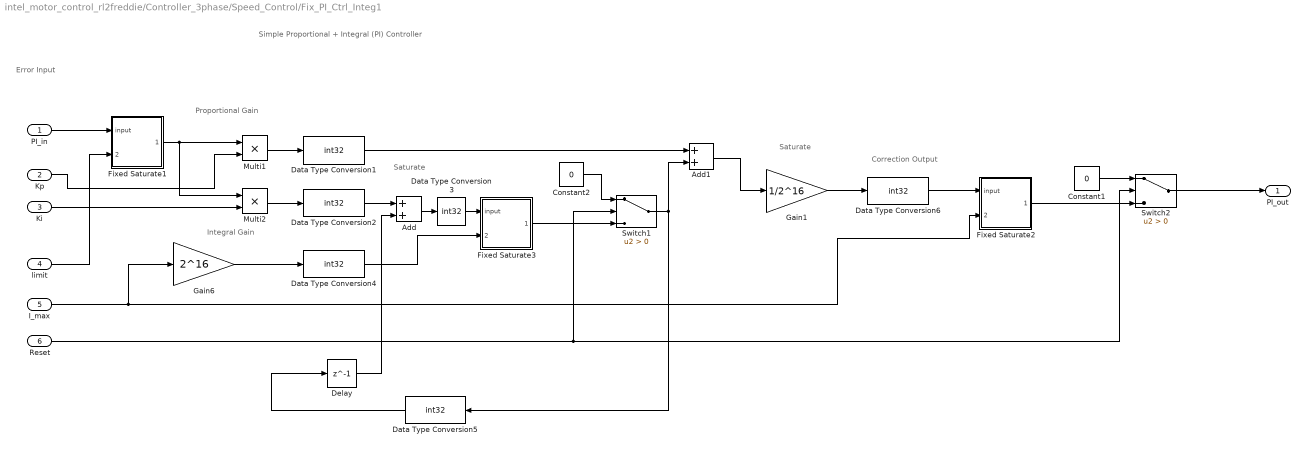
== system intel_motor_control_rl2freddie/Controller_3phase/Speed_Control/Fix_PI_Ctrl_Integ1 ==
  note: Correction Output
  note: Saturate
  note: Saturate
  note: Integral Gain
  note: Proportional Gain
  note: Error Input
  note: Simple Proportional + Integral (PI) Controller
  PI_in : Inport
  Kp : Inport  Port=2
  Ki : Inport  Port=3
  limit : Inport  Port=4
  I_max : Inport  Port=5
  Reset : Inport  Port=6
  Add : Sum
  Add1 : Sum
  Constant1 : Constant  Value=0  OutDataTypeStr=Inherit: Inherit via back propagation
  Constant2 : Constant  Value=0  OutDataTypeStr=Inherit: Inherit via back propagation
  Data Type Conversion{1..6} (6 alike) : DataTypeConversion  OutDataTypeStr=int32
  Delay : Delay  DelayLength=1  InitialCondition=0
  Fixed Saturate1 : Subsystem
  Fixed Saturate2 : Subsystem
  Fixed Saturate3 : Subsystem
  Gain1 : Gain  Gain=1/2^16
  Gain6 : Gain  Gain=2^16
  Multi1 : Product  Inputs=**  RndMeth=Zero  SaturateOnIntegerOverflow=on
  Multi2 : Product  Inputs=**  RndMeth=Zero  SaturateOnIntegerOverflow=on
  Switch1 : Switch  Criteria=u2 > Threshold
  Switch2 : Switch  Criteria=u2 > Threshold
  PI_out : Outport
  wires:
  Switch1/1 -> Add1/2, Data Type Conversion5/1
  Fixed Saturate3/1(output) -> Switch1/3
  Constant2/1 -> Switch1/1
  Constant1/1 -> Switch2/1
  Reset/1 -> Switch2/2, Switch1/2
  Switch2/1 -> PI_out/1
  Fixed Saturate2/1(output) -> Switch2/3
  Data Type Conversion6/1 -> Fixed Saturate2/1(input)
  Data Type Conversion5/1 -> Delay/1
  Data Type Conversion3/1 -> Fixed Saturate3/1(input)
  Data Type Conversion2/1 -> Add/1
  Data Type Conversion1/1 -> Add1/1
  Data Type Conversion4/1 -> Fixed Saturate3/2(abs_max)
  Gain1/1 -> Data Type Conversion6/1
  Gain6/1 -> Data Type Conversion4/1
  limit/1 -> Fixed Saturate1/2(abs_max)
  PI_in/1 -> Fixed Saturate1/1(input)
  Fixed Saturate1/1(output) -> Multi2/1, Multi1/1
  Delay/1 -> Add/2
  Add/1 -> Data Type Conversion3/1
  Add1/1 -> Gain1/1
  Multi1/1 -> Data Type Conversion1/1
  Multi2/1 -> Data Type Conversion2/1
  I_max/1 -> Gain6/1, Fixed Saturate2/2(abs_max)
  Kp/1 -> Multi1/2
  Ki/1 -> Multi2/2

== system intel_motor_control_rl2freddie/Controller_3phase/Speed_Control/Speed Filter ==
  Velocity : Inport
  Ks : Inport  Port=2
  Add : Sum  Inputs=-+
  Constant6 : Constant  OutDataTypeStr=Inherit: Inherit via back propagation
  Data Type Conversion1 : DataTypeConversion  OutDataTypeStr=int32
  Data Type Conversion4 : DataTypeConversion  OutDataTypeStr=int32
  Delay1 : Delay  DelayLength=1  InitialCondition=0
  Multi1 : Product  Inputs=**  RndMeth=Zero  SaturateOnIntegerOverflow=on
  Multi2 : Product  Inputs=**  RndMeth=Zero  SaturateOnIntegerOverflow=on
  Sum : Sum  Inputs=|++
  Speed : Outport
  wires:
  Add/1 -> Multi1/1
  Constant6/1 -> Add/2
  Ks/1 -> Multi2/2, Add/1
  Multi1/1 -> Sum/2
  Sum/1 -> Data Type Conversion4/1, Data Type Conversion1/1  "VelocityFiltered"
  Multi2/1 -> Sum/1
  Delay1/1 -> Multi1/2  "VelocityFilteredPrevious"
  Velocity/1 -> Multi2/1  "VelocityRaw"
  Data Type Conversion4/1 -> Delay1/1
  Data Type Conversion1/1 -> Speed/1

== system intel_motor_control_rl2freddie/Controller_equiv_DC_motor1/PI_Ctrl_float_speed/Reinforcement Learning1 ==
  speederror : Inport
  isdone : Inport  Port=2
  energy measure : Inport  Port=3
  speedfb : Inport  Port=4
  cfb : Inport  Port=5
  prevact : Inport  Port=6
  abslimit : Inport  Port=7
  speedin : Inport  Port=8
  Abs : Abs
  Add : Sum
  Delay : Delay  DelayLength=1
  Display : Display
  GreaterThan : RelationalOperator  Operator=>  OutDataTypeStr=boolean  RndMeth=Simplest
  Multiply : Gain
  Observations : Subsystem
  RL Agent : rllib/RL Agent  Agent=agent  ExternalActionAsInput=off  ProvideCumRwd=off  TreatAsDirectFeedthrough=on
  Reward : Subsystem  Commented=on
  Reward1 : Subsystem  Commented=on
  Subsystem : Subsystem
  action : Outport
  wires:
  Observations/1(observations) -> RL Agent/1
  isdone/1 -> RL Agent/3
  speederror/1 -> Subsystem/3(speed_error), Observations/1(speed err)
  speedfb/1 -> Observations/2(speedfb)
  cfb/1 -> Subsystem/2(current), Observations/3(curfb)
  Add/1 -> Delay/1, action/1
  RL Agent/1 -> Display/1, Add/1
  Delay/1 -> Subsystem/1(action), Observations/6(prevact), Abs/1
  abslimit/1 -> GreaterThan/2
  Abs/1 -> GreaterThan/1
  GreaterThan/1 -> Observations/4(lim)
  speedin/1 -> Observations/5(speedin)
  Multiply/1 -> Add/2
  prevact/1 -> Multiply/1
  Subsystem/1(Out1) -> RL Agent/2

== system intel_motor_control_rl2freddie/Controller_equiv_DC_motor1/PI_Ctrl_float_speed/limit_abs_value_of_output ==
  input : Inport
  abs_max : Inport  Port=2
  CmpLT : RelationalOperator  Operator=<  OutDataTypeStr=boolean  RndMeth=Nearest
  CmpLT1 : RelationalOperator  OutDataTypeStr=boolean  RndMeth=Nearest
  Switch : Switch  Criteria=u2 ~= 0  Threshold=Position_PI_Limit  ZeroCross=off
  Switch1 : Switch  Criteria=u2 ~= 0  Threshold=I_max  ZeroCross=off
  Unary Minus : UnaryMinus
  output : Outport
  wires:
  Unary Minus/1 -> CmpLT/2, Switch1/1
  Switch1/1 -> output/1
  Switch/1 -> Switch1/3
  CmpLT/1 -> Switch1/2
  input/1 -> CmpLT/1, Switch/3, CmpLT1/1
  abs_max/1 -> Unary Minus/1, CmpLT1/2, Switch/1
  CmpLT1/1 -> Switch/2

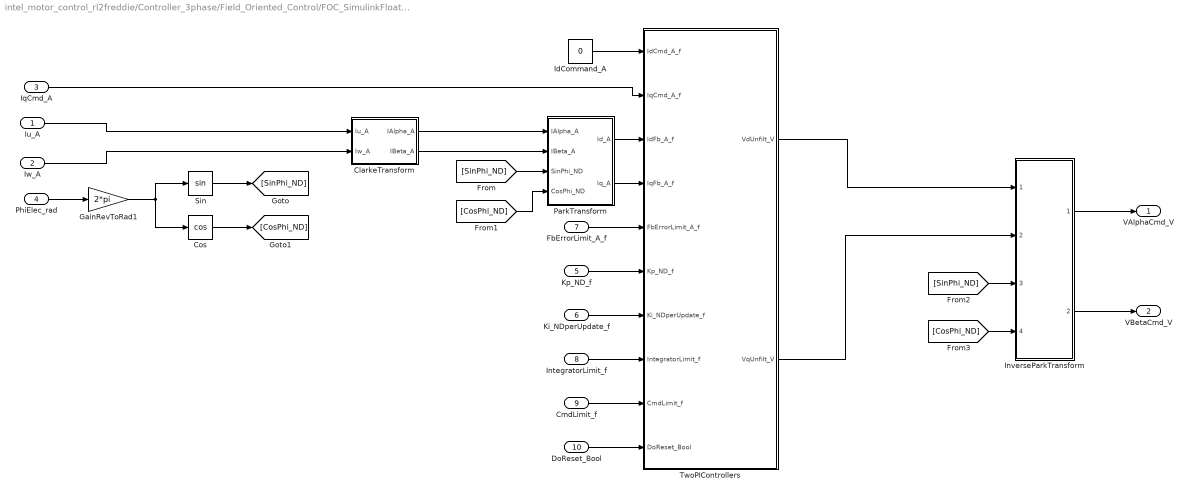
== system intel_motor_control_rl2freddie/Controller_3phase/Field_Oriented_Control/FOC_SimulinkFloat/FOC_Simulink_float ==
  Iu_A : Inport
  Iw_A : Inport  Port=2
  IqCmd_A : Inport  Port=3
  PhiElec_rad : Inport  Port=4
  Kp_ND_f : Inport  Port=5
  Ki_NDperUpdate_f : Inport  Port=6
  FbErrorLimit_A_f : Inport  Port=7
  IntegratorLimit_f : Inport  Port=8
  CmdLimit_f : Inport  Port=9
  DoReset_Bool : Inport  Port=10
  ClarkeTransform : Subsystem
  Cos : Trigonometry  Operator=cos
  GainRevToRad1 : Gain  Gain=2*pi
  IdCommand_A : Constant  Value=0
  InverseParkTransform : Subsystem
  ParkTransform : Subsystem
  Sin : Trigonometry
  TwoPIControllers : Subsystem
  VAlphaCmd_V : Outport
  VBetaCmd_V : Outport  Port=2
  wires:
  GainRevToRad1/1 -> Cos/1, Sin/1
  IqCmd_A/1 -> TwoPIControllers/2(IqCmd_A_f)
  Iu_A/1 -> ClarkeTransform/1(Iu_A)
  Iw_A/1 -> ClarkeTransform/2(Iw_A)
  ClarkeTransform/2(IBeta_A) -> ParkTransform/2(IBeta_A)
  ClarkeTransform/1(IAlpha_A) -> ParkTransform/1(IAlpha_A)
  PhiElec_rad/1 -> GainRevToRad1/1
  ParkTransform/1(Id_A) -> TwoPIControllers/3(IdFb_A_f)
  IdCommand_A/1 -> TwoPIControllers/1(IdCmd_A_f)
  ParkTransform/2(Iq_A) -> TwoPIControllers/4(IqFb_A_f)
  [SinPhi_ND] -> ParkTransform/3(SinPhi_ND)
  [CosPhi_ND] -> ParkTransform/4(CosPhi_ND)
  TwoPIControllers/2(VqUnfilt_V) -> InverseParkTransform/2(VqCmd_V)
  Sin/1 -> [SinPhi_ND]
  Cos/1 -> [CosPhi_ND]
  TwoPIControllers/1(VdUnfilt_V) -> InverseParkTransform/1(VdCmd_V)
  DoReset_Bool/1 -> TwoPIControllers/10(DoReset_Bool)
  [SinPhi_ND] -> InverseParkTransform/3(SinPhi_ND)
  [CosPhi_ND] -> InverseParkTransform/4(CosPhi_ND)
  CmdLimit_f/1 -> TwoPIControllers/9(CmdLimit_f)
  IntegratorLimit_f/1 -> TwoPIControllers/8(IntegratorLimit_f)
  Ki_NDperUpdate_f/1 -> TwoPIControllers/7(Ki_NDperUpdate_f)
  Kp_ND_f/1 -> TwoPIControllers/6(Kp_ND_f)
  InverseParkTransform/2(VBetaCmd_V) -> VBetaCmd_V/1
  FbErrorLimit_A_f/1 -> TwoPIControllers/5(FbErrorLimit_A_f)
  InverseParkTransform/1(VAlphaCmd_V) -> VAlphaCmd_V/1

== system intel_motor_control_rl2freddie/Controller_3phase/Speed_Control/Fix_PI_Ctrl_Integ1/Fixed Saturate1 ==
  input : Inport
  abs_max : Inport  Port=2
  CmpLT : RelationalOperator  Operator=<  OutDataTypeStr=boolean  RndMeth=Nearest
  CmpLT1 : RelationalOperator  OutDataTypeStr=boolean  RndMeth=Nearest
  Switch : Switch  Criteria=u2 ~= 0  Threshold=Position_PI_Limit  ZeroCross=off
  Switch1 : Switch  Criteria=u2 ~= 0  Threshold=I_max  ZeroCross=off
  Unary Minus : UnaryMinus
  output : Outport
  wires:
  CmpLT1/1 -> Switch/2
  abs_max/1 -> Switch/1, CmpLT1/2, Unary Minus/1
  input/1 -> CmpLT1/1, Switch/3, CmpLT/1
  CmpLT/1 -> Switch1/2
  Switch/1 -> Switch1/3
  Switch1/1 -> output/1
  Unary Minus/1 -> Switch1/1, CmpLT/2

== system intel_motor_control_rl2freddie/Controller_3phase/Speed_Control/Fix_PI_Ctrl_Integ1/Fixed Saturate2 ==
  input : Inport
  abs_max : Inport  Port=2
  CmpLT : RelationalOperator  Operator=<  OutDataTypeStr=boolean  RndMeth=Nearest
  CmpLT1 : RelationalOperator  OutDataTypeStr=boolean  RndMeth=Nearest
  Switch : Switch  Criteria=u2 ~= 0  Threshold=Position_PI_Limit  ZeroCross=off
  Switch1 : Switch  Criteria=u2 ~= 0  Threshold=I_max  ZeroCross=off
  Unary Minus : UnaryMinus
  output : Outport
  wires:
  CmpLT1/1 -> Switch/2
  abs_max/1 -> Switch/1, CmpLT1/2, Unary Minus/1
  input/1 -> CmpLT1/1, Switch/3, CmpLT/1
  CmpLT/1 -> Switch1/2
  Switch/1 -> Switch1/3
  Switch1/1 -> output/1
  Unary Minus/1 -> Switch1/1, CmpLT/2

== system intel_motor_control_rl2freddie/Controller_3phase/Speed_Control/Fix_PI_Ctrl_Integ1/Fixed Saturate3 ==
  input : Inport
  abs_max : Inport  Port=2
  CmpLT : RelationalOperator  Operator=<  OutDataTypeStr=boolean  RndMeth=Nearest
  CmpLT1 : RelationalOperator  OutDataTypeStr=boolean  RndMeth=Nearest
  Switch : Switch  Criteria=u2 ~= 0  Threshold=Position_PI_Limit  ZeroCross=off
  Switch1 : Switch  Criteria=u2 ~= 0  Threshold=I_max  ZeroCross=off
  Unary Minus : UnaryMinus
  output : Outport
  wires:
  Unary Minus/1 -> CmpLT/2, Switch1/1
  Switch1/1 -> output/1
  Switch/1 -> Switch1/3
  CmpLT/1 -> Switch1/2
  input/1 -> CmpLT/1, Switch/3, CmpLT1/1
  abs_max/1 -> Unary Minus/1, CmpLT1/2, Switch/1
  CmpLT1/1 -> Switch/2

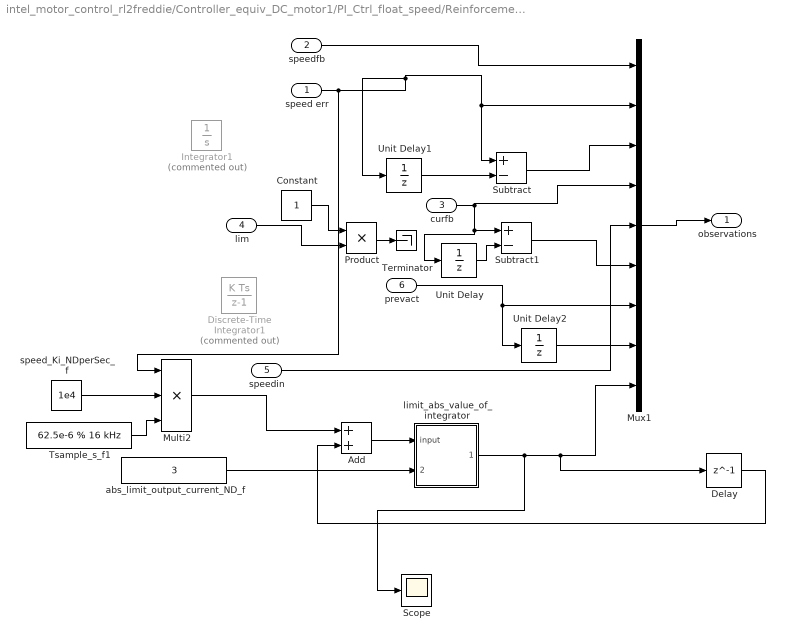
== system intel_motor_control_rl2freddie/Controller_equiv_DC_motor1/PI_Ctrl_float_speed/Reinforcement Learning1/Observations ==
  speed err : Inport
  speedfb : Inport  Port=2
  curfb : Inport  Port=3
  lim : Inport  Port=4
  speedin : Inport  Port=5
  prevact : Inport  Port=6
  Add : Sum
  Constant : Constant
  Delay : Delay  DelayLength=1  InitialCondition=0
  Discrete-Time Integrator1 : DiscreteIntegrator  Commented=on  SampleTime=-1  ICPrevOutput=DiscIntNeverNeededParam  ICPrevScaledInput=DiscIntNeverNeededParam
  Integrator1 : Integrator  Commented=on
  Multi2 : Product  Inputs=***  RndMeth=Zero  SaturateOnIntegerOverflow=on
  Mux1 : Mux  Inputs=9
  Product : Product
  Scope : Scope
  Subtract : Sum  Inputs=+-
  Subtract1 : Sum  Inputs=+-
  Terminator : Terminator
  Tsample_s_f1 : Constant  Value=62.5e-6 % 16 kHz  OutDataTypeStr=double
  Unit Delay : UnitDelay  SampleTime=-1  HasFrameUpgradeWarning=on
  Unit Delay1 : UnitDelay  SampleTime=-1  HasFrameUpgradeWarning=on
  Unit Delay2 : UnitDelay  SampleTime=-1  HasFrameUpgradeWarning=on
  abs_limit_output_current_ND_f : Constant  Value=3  OutDataTypeStr=double
  limit_abs_value_of_integrator : Subsystem
  speed_Ki_NDperSec_f : Constant  Value=1e4  OutDataTypeStr=double
  observations : Outport  VectorParamsAs1DForOutWhenUnconnected=off
  wires:
  Mux1/1 -> observations/1
  speedfb/1 -> Mux1/1
  curfb/1 -> Subtract1/1, Unit Delay/1, Mux1/4
  Unit Delay1/1 -> Subtract/2
  Subtract/1 -> Mux1/3
  lim/1 -> Product/2
  Constant/1 -> Product/1
  prevact/1 -> Unit Delay2/1, Mux1/7
  speedin/1 -> Mux1/5
  Product/1 -> Terminator/1
  Unit Delay/1 -> Subtract1/2
  Subtract1/1 -> Mux1/6
  Unit Delay2/1 -> Mux1/8
  limit_abs_value_of_integrator/1(output) -> Scope/1, Delay/1, Mux1/9
  Delay/1 -> Add/2
  abs_limit_output_current_ND_f/1 -> limit_abs_value_of_integrator/2(abs_max)
  Add/1 -> limit_abs_value_of_integrator/1(input)
  speed err/1 -> Multi2/1, Subtract/1, Mux1/2, Unit Delay1/1
  speed_Ki_NDperSec_f/1 -> Multi2/2
  Tsample_s_f1/1 -> Multi2/3
  Multi2/1 -> Add/1

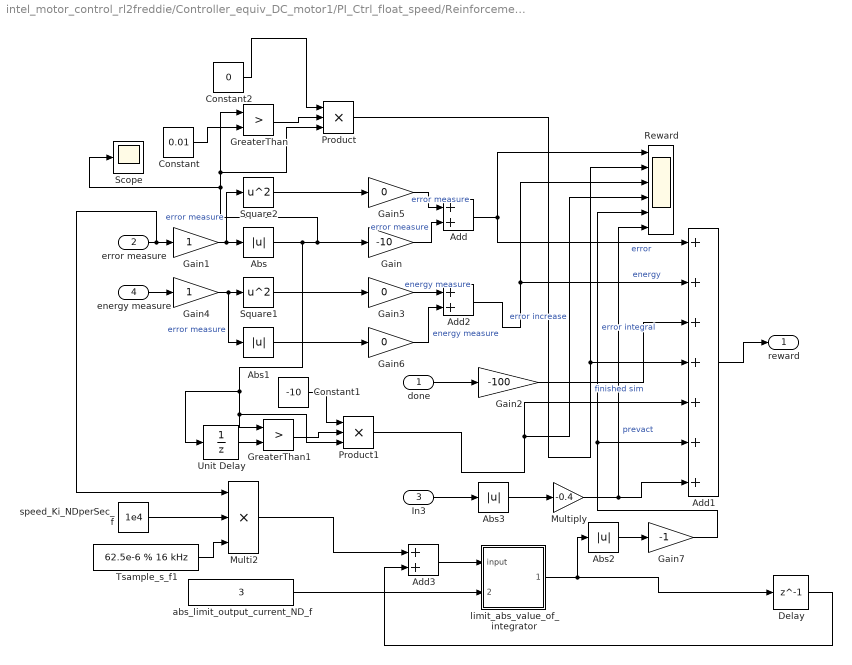
== system intel_motor_control_rl2freddie/Controller_equiv_DC_motor1/PI_Ctrl_float_speed/Reinforcement Learning1/Reward ==
  done : Inport
  error measure : Inport  Port=2
  In3 : Inport  Port=3
  energy measure : Inport  Port=4
  Abs{,1..3} (4 alike) : Abs
  Add : Sum
  Add1 : Sum  Inputs=+++++++
  Add2 : Sum
  Add3 : Sum
  Constant : Constant  Value=0.01
  Constant1 : Constant  Value=-10
  Constant2 : Constant  Value=0
  Delay : Delay  DelayLength=1  InitialCondition=0
  Gain : Gain  Gain=-10
  Gain1 : Gain
  Gain2 : Gain  Gain=-100
  Gain3 : Gain  Gain=0
  Gain4 : Gain
  Gain5 : Gain  Gain=0
  Gain6 : Gain  Gain=0
  Gain7 : Gain  Gain=-1
  GreaterThan : RelationalOperator  Operator=>  OutDataTypeStr=boolean  RndMeth=Simplest
  GreaterThan1 : RelationalOperator  Operator=>  OutDataTypeStr=boolean  RndMeth=Simplest
  Multi2 : Product  Inputs=***  RndMeth=Zero  SaturateOnIntegerOverflow=on
  Multiply : Gain  Gain=-0.4
  Product : Product  Inputs=3
  Product1 : Product  Inputs=3
  Reward : Scope  NumInputPorts=6
  Scope : Scope
  Square1 : Math  Operator=square  SaturateOnIntegerOverflow=on
  Square2 : Math  Operator=square  SaturateOnIntegerOverflow=on
  Tsample_s_f1 : Constant  Value=62.5e-6 % 16 kHz  OutDataTypeStr=double
  Unit Delay : UnitDelay  SampleTime=-1  HasFrameUpgradeWarning=on
  abs_limit_output_current_ND_f : Constant  Value=3  OutDataTypeStr=double
  limit_abs_value_of_integrator : Subsystem
  speed_Ki_NDperSec_f : Constant  Value=1e4  OutDataTypeStr=double
  reward : Outport  VectorParamsAs1DForOutWhenUnconnected=off
  wires:
  Add1/1 -> reward/1
  Gain2/1 -> Add1/3  "finished sim"
  done/1 -> Gain2/1
  Gain/1 -> Add/2  "error measure"
  Square1/1 -> Gain3/1
  error measure/1 -> Multi2/1, Gain1/1
  energy measure/1 -> Gain4/1
  Gain4/1 -> Abs1/1, Square1/1  "error measure"
  Gain1/1 -> Square2/1, Abs/1  "error measure"
  Square2/1 -> Gain5/1
  Gain5/1 -> Add/1  "error measure"
  Add/1 -> Reward/1, Add1/1  "error"
  Add2/1 -> Reward/3, Add1/2  "energy"
  Abs1/1 -> Gain6/1
  Gain6/1 -> Add2/2  "energy measure"
  Gain3/1 -> Add2/1  "energy measure"
  Constant/1 -> GreaterThan/2
  GreaterThan/1 -> Product/2
  Product/1 -> Reward/2, Add1/4
  Constant2/1 -> Product/1
  Constant1/1 -> Product1/1
  GreaterThan1/1 -> Product1/2
  Abs/1 -> Unit Delay/1, Product1/3, GreaterThan1/1, Scope/1, Product/3, GreaterThan/1, Gain/1
  Unit Delay/1 -> GreaterThan1/2
  Product1/1 -> Reward/4, Add1/5  "error increase"
  Tsample_s_f1/1 -> Multi2/3
  speed_Ki_NDperSec_f/1 -> Multi2/2
  Delay/1 -> Add3/2
  Add3/1 -> limit_abs_value_of_integrator/1(input)
  Multi2/1 -> Add3/1
  abs_limit_output_current_ND_f/1 -> limit_abs_value_of_integrator/2(abs_max)
  limit_abs_value_of_integrator/1(output) -> Abs2/1, Delay/1
  Abs2/1 -> Gain7/1
  Gain7/1 -> Reward/5, Add1/6  "error integral"
  In3/1 -> Abs3/1
  Abs3/1 -> Multiply/1
  Multiply/1 -> Reward/6, Add1/7  "prevact"

== system intel_motor_control_rl2freddie/Controller_equiv_DC_motor1/PI_Ctrl_float_speed/Reinforcement Learning1/Reward1 ==
  done : Inport
  error measure : Inport  Port=2
  energy measure : Inport  Port=3
  Abs : Abs
  Abs1 : Abs
  Add : Sum
  Add1 : Sum  Inputs=+++
  Add2 : Sum
  Gain : Gain  Gain=-5
  Gain1 : Gain
  Gain2 : Gain  Gain=-100
  Gain3 : Gain  Gain=0
  Gain4 : Gain
  Gain5 : Gain  Gain=0
  Gain6 : Gain  Gain=0
  Reward : Scope  NumInputPorts=2
  Square1 : Math  Operator=square  SaturateOnIntegerOverflow=on
  Square2 : Math  Operator=square  SaturateOnIntegerOverflow=on
  reward : Outport  VectorParamsAs1DForOutWhenUnconnected=off
  wires:
  Add1/1 -> reward/1
  Gain2/1 -> Add1/3  "finished sim"
  done/1 -> Gain2/1
  Gain/1 -> Add/2  "error measure"
  Abs/1 -> Gain/1
  Square1/1 -> Gain3/1
  error measure/1 -> Gain1/1
  energy measure/1 -> Gain4/1
  Gain4/1 -> Abs1/1, Square1/1  "error measure"
  Gain1/1 -> Square2/1, Abs/1  "error measure"
  Square2/1 -> Gain5/1
  Gain5/1 -> Add/1  "error measure"
  Add/1 -> Reward/1, Add1/1  "error"
  Add2/1 -> Reward/2, Add1/2  "energy"
  Abs1/1 -> Gain6/1
  Gain6/1 -> Add2/2  "energy measure"
  Gain3/1 -> Add2/1  "energy measure"
